simulink model "gm_sampleModel1810_sub"  (R2023a)
settings: Solver=VariableStepAuto  StartTime=0.0  StopTime=10.0  RelTol=1e-3
libraries: simulink x4, hdlsllib x2
settings Model: Creator=user1  LastModifiedBy=user1
settings OptimizationCC: BlockReduction=off  ConditionallyExecuteInputs=off
settings DebuggingCC: InheritedTsInSrcMsg=none

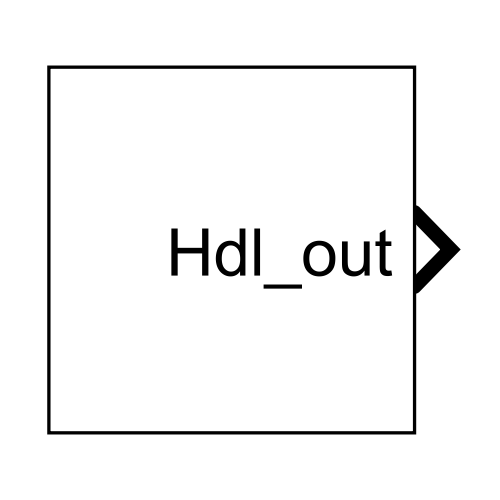
[thumbnail: Simulink's stored preview of the top-level diagram]
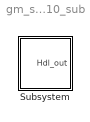
== system gm_sampleModel1810_sub ==
  Subsystem : Subsystem

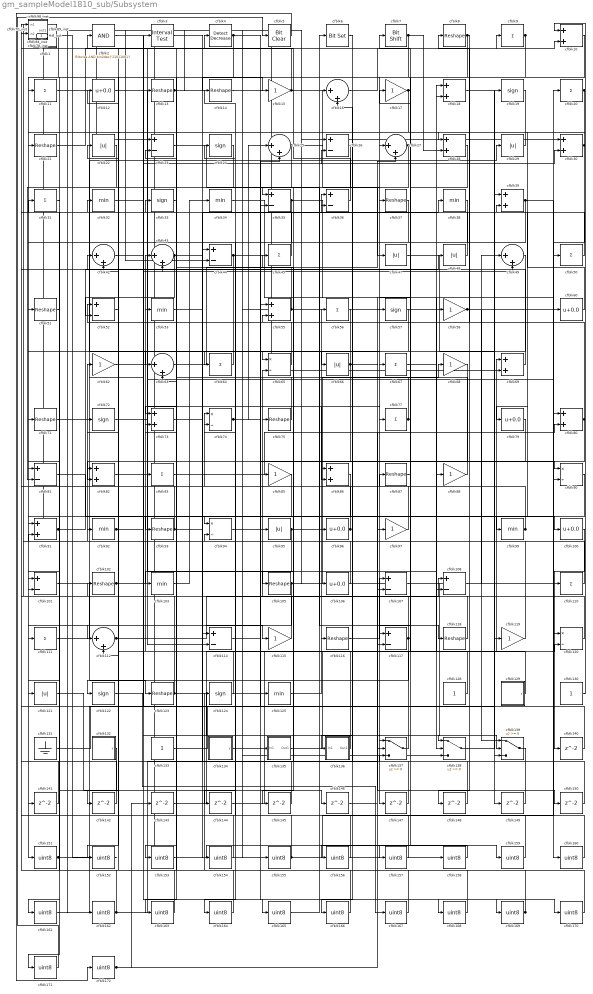
== system gm_sampleModel1810_sub/Subsystem ==
  cfblk1 : Subsystem  mask(Detect Rise Nonnegative){vinit=double(0), InputProcessing=Elements as channels (sample based), OutDataTypeStr=uint8}
      mask prompts: vinit "Simulink:masks:InitialCondition_MP"; InputProcessing "Simulink:masks:InputProcessing_MP"; OutDataTypeStr "Simulink:masks:OutputDataType_MP"
      mask help: Simulink:masks:DetectRiseNonnegative_MD
      mask init:
      | InputProcessing = 'Elements as channels (sample based)';
      | OutDataTypeStr = 'uint8';
      | vinit = double(0);
      mask TypeOptions InputProcessing: Simulink:masks:ColumnsAsChannelsFrameBased | Simulink:masks:ElementsAsChannelsSampleBased
      mask TypeOptions OutDataTypeStr: Simulink:masks:uint8 | Simulink:masks:boolean
      mask Display: fprintf('U >= 0\n&  NOT\nU/z >= 0')
  cfblk{10,18,28,30,39,55,69,73,80,82,86,91} (12 alike) : Sum  OutDataTypeStr=uint8
  cfblk{12,60,79,96,100,106} (6 alike) : Bias  Bias=0.0  SaturateOnIntegerOverflow=off
  cfblk{23,26,35..36,44,52,81,101,107..108,114,117} (12 alike) : Sum  Inputs=+-  OutDataTypeStr=uint8
  cfblk{8,13..14,21,37,51,71,75,87,93,102,105,116,118,123} (15 alike) : Reshape
  cfblk{32,34,38,53,92,99,103,125} (8 alike) : MinMax  OutDataTypeStr=uint8
  cfblk{9,11,20,31,45,50,56,64,67,77,83,110..111} (13 alike) : Sum  Inputs=+  OutDataTypeStr=uint8
  cfblk{16,25,27,42..43,49,63,112} (8 alike) : Sum  Inputs=|++  OutDataTypeStr=uint8
  cfblk113_inst : Subsystem
  cfblk{15,17,58,62,68,85,88,97,115,119} (10 alike) : Gain  OutDataTypeStr=uint8
  cfblk{65,74,90,94,120} (5 alike) : Product  Inputs=*/  OutDataTypeStr=uint8  RndMeth=Zero  SaturateOnIntegerOverflow=on
  cfblk{22,29,47..48,66,95,121} (7 alike) : Abs  OutDataTypeStr=uint8  SaturateOnIntegerOverflow=off
  cfblk{19,24,33,57,72,122,124} (7 alike) : Signum
  cfblk128 : Constant  OutDataTypeStr=uint8  SampleTime=-1
  cfblk129 : Subsystem  mask(Counter Limited){uplimit=double(7), tsamp=double(-1)}
      mask prompts: uplimit "Simulink:masks:UpperLimit_MP"; tsamp "Simulink:masks:SampleTime_MP"
      mask help: Simulink:masks:CounterLimited_MD
      mask init:
      | nbits = double(8);
      | tsamp = double(-1);
      | uplimit = double(7);
  cfblk130 : Constant  OutDataTypeStr=uint8  SampleTime=-1
  cfblk131 : Ground
  cfblk132 : Subsystem  mask(Counter Free-Running){NumBits=double(16), tsamp=double(-1)}
      mask prompts: NumBits "Simulink:masks:NumberOfBits_MP"; tsamp "Simulink:masks:SampleTime_MP"
      mask help: Simulink:masks:CounterFreeRunning_MD
  cfblk133 : Constant  OutDataTypeStr=uint8  SampleTime=-1
  cfblk134 : Subsystem  mask(Counter Limited){uplimit=double(7), tsamp=double(-1)}
      mask prompts: uplimit "Simulink:masks:UpperLimit_MP"; tsamp "Simulink:masks:SampleTime_MP"
      mask help: Simulink:masks:CounterLimited_MD
      mask init:
      | nbits = double(8);
      | tsamp = double(-1);
      | uplimit = double(7);
  cfblk135 : Subsystem
  cfblk136 : Subsystem
  cfblk137 : Switch  OutDataTypeStr=uint8  SaturateOnIntegerOverflow=off  InputSameDT=off
  cfblk138 : Switch  OutDataTypeStr=uint8  SaturateOnIntegerOverflow=off  InputSameDT=off
  cfblk139 : Switch  OutDataTypeStr=uint8  SaturateOnIntegerOverflow=off  InputSameDT=off
  cfblk{140..150} (11 alike) : Delay  SampleTime=1
  cfblk{151..172} (22 alike) : DataTypeConversion  OutDataTypeStr=uint8  SaturateOnIntegerOverflow=off  RndMeth=Floor
  cfblk2 : simulink/Logic and Bit Operations/Bitwise Operator  logicop=AND  UseBitMask=on  BitMask=bin2dec('11011001')  BitMaskRealWorld=Stored Integer
      settings: LibrarySourceBlock=|
      | hdlsllib/Logic and Bit
      | Operations/Bitwise
      | Operator
  cfblk3 : hdlsllib/Logic and Bit Operations/Interval Test  IntervalClosedRight=on  uplimit=0.5  IntervalClosedLeft=on  lowlimit=-0.5  OutDataTypeStr=uint8
  cfblk4 : simulink/Logic and Bit Operations/Detect Decrease  vinit=0.0  OutDataTypeStr=uint8
      settings: LibrarySourceBlock=|
      | hdlsllib/Logic and Bit
      | Operations/Detect
      | Decrease
  cfblk41_inst : Subsystem
  cfblk46_inst : Subsystem
  cfblk5 : simulink/Logic and Bit Operations/Bit Clear  iBit=0
      settings: LibrarySourceBlock=|
      | hdlsllib/Logic and Bit
      | Operations/Bit Clear
  cfblk54_inst : Subsystem
  cfblk59_inst : Subsystem
  cfblk6 : simulink/Logic and Bit Operations/Bit Set  iBit=0
      settings: LibrarySourceBlock=|
      | hdlsllib/Logic and Bit
      | Operations/Bit Set
  cfblk61_inst : Subsystem
  cfblk7 : hdlsllib/Logic and Bit Operations/Bit Shift  mode=Shift Left Logical  N=0
  cfblk70_inst : Subsystem
  cfblk78_inst : Subsystem
  cfblk84_inst : Subsystem
  cfblk89_inst : Subsystem
  cfblk98_inst : Subsystem
  Hdl_out : Outport  OutDataTypeStr=uint8  SampleTime=1
  wires:
  cfblk1/1(Y) -> cfblk151/1
  cfblk10/1 -> cfblk147/1
  cfblk100/1 -> cfblk140/1
  cfblk101/1 -> cfblk123/1
  cfblk102/1 -> cfblk114/2, cfblk10/2
  cfblk103/1 -> cfblk34/1
  cfblk105/1 -> cfblk68/1, cfblk141/1
  cfblk106/1 -> cfblk84_inst/1(in1)
  cfblk107/1 -> cfblk139/2
  cfblk108/1 -> cfblk49/1
  cfblk11/1 -> cfblk67/1
  cfblk110/1 -> cfblk65/2
  cfblk111/1 -> cfblk29/1
  cfblk112/1 -> cfblk108/1, cfblk115/1
  cfblk113_inst/1(out1) -> cfblk44/2, cfblk138/3
  cfblk114/1 -> cfblk120/2
  cfblk115/1 -> cfblk14/1
  cfblk116/1 -> cfblk107/1
  cfblk117/1 -> cfblk78_inst/1(in1), cfblk122/1
  cfblk118/1 -> cfblk113_inst/1(in1)
  cfblk119/1 -> cfblk62/1
  cfblk12/1 -> cfblk107/2
  cfblk120/1 -> cfblk75/1
  cfblk121/1 -> cfblk146/1
  cfblk122/1 -> cfblk167/1
  cfblk123/1 -> cfblk78_inst/2(in2), cfblk139/3, cfblk138/1
  cfblk124/1 -> cfblk43/1
  cfblk125/1 -> cfblk56/1
  cfblk128/1 -> cfblk17/1
  cfblk129/1(y) -> cfblk92/1
  cfblk13/1 -> cfblk15/1, cfblk77/1
  cfblk130/1 -> cfblk10/1
  cfblk131/1 -> cfblk25/2
  cfblk132/1(y) -> cfblk161/1
  cfblk133/1 -> cfblk19/1
  cfblk134/1(y) -> cfblk116/1
  cfblk135/1(Out1) -> cfblk18/2
  cfblk136/1(Out1) -> cfblk74/1
  cfblk137/1 -> cfblk53/1
  cfblk138/1 -> cfblk120/1
  cfblk139/1 -> cfblk137/3
  cfblk14/1 -> cfblk90/1
  cfblk140/1 -> cfblk84_inst/2(in2)
  cfblk141/1 -> cfblk70_inst/2(in2)
  cfblk142/1 -> cfblk46_inst/2(in2)
  cfblk143/1 -> cfblk69/1
  cfblk144/1 -> cfblk39/1
  cfblk145/1 -> cfblk52/1
  cfblk146/1 -> cfblk80/2
  cfblk147/1 -> cfblk55/2
  cfblk148/1 -> cfblk16/2
  cfblk149/1 -> cfblk36/1
  cfblk15/1 -> cfblk59_inst/2(in2), cfblk37/1
  cfblk150/1 -> cfblk44/1
  cfblk151/1 -> cfblk106/1, cfblk3/1
  cfblk152/1 -> cfblk1/1(U)
  cfblk153/1 -> cfblk159/1
  cfblk154/1 -> cfblk33/1
  cfblk155/1 -> cfblk94/2, cfblk50/1
  cfblk156/1 -> cfblk61_inst/1(in1)
  cfblk157/1 -> cfblk61_inst/2(in2)
  cfblk158/1 -> cfblk156/1
  cfblk159/1 -> cfblk54_inst/1(in1)
  cfblk16/1 -> cfblk9/1
  cfblk160/1 -> cfblk54_inst/2(in2)
  cfblk161/1 -> cfblk95/1
  cfblk162/1 -> cfblk98_inst/2(in2), cfblk91/2, cfblk137/2, cfblk31/1
  cfblk163/1 -> cfblk89_inst/1(in1)
  cfblk164/1 -> cfblk89_inst/2(in2)
  cfblk165/1 -> cfblk6/1
  cfblk166/1 -> cfblk124/1
  cfblk167/1 -> cfblk2/1
  cfblk168/1 -> cfblk102/1
  cfblk169/1 -> cfblk73/2, cfblk22/1
  cfblk17/1 -> cfblk93/1, cfblk157/1
  cfblk170/1 -> cfblk32/1
  cfblk171/1 -> cfblk5/1
  cfblk172/1 -> cfblk117/2, cfblk143/1
  cfblk18/1 -> cfblk149/1
  cfblk19/1 -> cfblk28/1
  cfblk2/1 -> cfblk168/1
  cfblk20/1 -> cfblk79/1, cfblk101/2
  cfblk21/1 -> cfblk4/1
  cfblk22/1 -> cfblk171/1
  cfblk23/1 -> cfblk96/1
  cfblk24/1 -> cfblk81/1
  cfblk25/1 -> cfblk81/2, cfblk47/1
  cfblk26/1 -> cfblk105/1
  cfblk27/1 -> cfblk35/1, cfblk112/2
  cfblk28/1 -> cfblk57/1
  cfblk29/1 -> cfblk21/1
  cfblk3/1 -> cfblk154/1
  cfblk30/1 -> cfblk27/1, cfblk90/2
  cfblk31/1 -> cfblk101/1
  cfblk32/1 -> cfblk169/1
  cfblk33/1 -> cfblk153/1
  cfblk34/1 -> cfblk97/1
  cfblk35/1 -> cfblk51/1, cfblk138/2
  cfblk36/1 -> cfblk46_inst/1(in1)
  cfblk37/1 -> cfblk103/1
  cfblk38/1 -> cfblk65/1
  cfblk39/1 -> cfblk80/1, cfblk94/1, cfblk99/1
  cfblk4/1 -> cfblk91/1, cfblk170/1
  cfblk41_inst/1(out1) -> cfblk13/1
  cfblk42/1 -> cfblk165/1
  cfblk43/1 -> cfblk52/2, cfblk108/2
  cfblk44/1 -> cfblk71/1, cfblk160/1
  cfblk45/1 -> cfblk59_inst/1(in1)
  cfblk46_inst/1(out1) -> cfblk69/2
  cfblk47/1 -> cfblk119/1
  cfblk48/1 -> cfblk12/1
  cfblk49/1 -> cfblk145/1
  cfblk5/1 -> cfblk172/1
  cfblk50/1 -> cfblk39/2
  cfblk51/1 -> cfblk121/1
  cfblk52/1 -> cfblk112/1
  cfblk53/1 -> cfblk114/1
  cfblk54_inst/1(out1) -> cfblk158/1
  cfblk55/1 -> cfblk41_inst/2(in2), cfblk118/1
  cfblk56/1 -> cfblk164/1
  cfblk57/1 -> cfblk66/1
  cfblk58/1 -> cfblk60/1, cfblk139/1
  cfblk59_inst/1(out1) -> cfblk125/1
  cfblk6/1 -> cfblk166/1
  cfblk60/1 -> cfblk36/2
  cfblk61_inst/1(out1) -> cfblk155/1
  cfblk62/1 -> cfblk86/2
  cfblk63/1 -> cfblk27/2
  cfblk64/1 -> cfblk63/1
  cfblk65/1 -> cfblk42/1
  cfblk66/1 -> cfblk82/2, cfblk150/1, cfblk64/1
  cfblk67/1 -> cfblk88/1
  cfblk68/1 -> cfblk142/1
  cfblk69/1 -> cfblk70_inst/1(in1)
  cfblk7/1 -> cfblk82/1, cfblk28/2
  cfblk70_inst/1(out1) -> cfblk23/1, cfblk16/1
  cfblk71/1 -> cfblk26/2
  cfblk72/1 -> cfblk20/1
  cfblk73/1 -> cfblk38/1
  cfblk74/1 -> cfblk35/2, cfblk25/1
  cfblk75/1 -> cfblk24/1
  cfblk77/1 -> cfblk23/2, cfblk113_inst/2(in2)
  cfblk78_inst/1(out1) -> cfblk98_inst/1(in1), cfblk110/1
  cfblk79/1 -> cfblk86/1
  cfblk8/1 -> cfblk117/1, cfblk148/1
  cfblk80/1 -> cfblk8/1, cfblk136/1(In1), cfblk45/1
  cfblk81/1 -> cfblk100/1
  cfblk82/1 -> cfblk135/1(In1)
  cfblk83/1 -> cfblk18/1
  cfblk84_inst/1(out1) -> cfblk58/1
  cfblk85/1 -> cfblk152/1
  cfblk86/1 -> cfblk111/1
  cfblk87/1 -> cfblk7/1
  cfblk88/1 -> cfblk55/1
  cfblk89_inst/1(out1) -> cfblk162/1
  cfblk9/1 -> cfblk73/1, cfblk11/1
  cfblk90/1 -> cfblk144/1
  cfblk91/1 -> cfblk48/1, Hdl_out/1
  cfblk92/1 -> cfblk72/1, cfblk49/2, cfblk43/2, cfblk137/1
  cfblk93/1 -> cfblk41_inst/1(in1), cfblk85/1
  cfblk94/1 -> cfblk26/1
  cfblk95/1 -> cfblk30/2, cfblk163/1
  cfblk96/1 -> cfblk63/2, cfblk74/2
  cfblk97/1 -> cfblk42/2
  cfblk98_inst/1(out1) -> cfblk30/1
  cfblk99/1 -> cfblk87/1, cfblk83/1

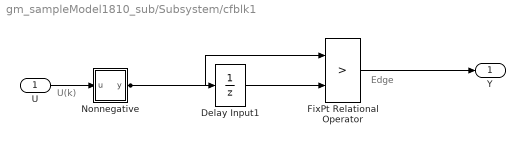
== system gm_sampleModel1810_sub/Subsystem/cfblk1 ==
  note: U(k)
  note: Edge
  U : Inport  OutDataTypeStr=uint8  SampleTime=1
  Delay Input1 : UnitDelay  Description=Store in Global RAM  DisableCoverage=on  InitialCondition=vinit  SampleTime=-1  HasFrameUpgradeWarning=on
  FixPt Relational Operator : RelationalOperator  Operator=>  OutDataTypeStr=fixdt(0, 8)  ZeroCross=off  InputSameDT=off
  Nonnegative : Subsystem  mask(Compare To Zero){relop=>=, OutDataTypeStr=boolean, ZeroCross=off}
      mask prompts: relop "Simulink:masks:Operator_MP"; OutDataTypeStr "Simulink:masks:OutputDataType_MP"; ZeroCross "Simulink:masks:EnableZerocrossingDetection_MP"
      mask help: Simulink:masks:CompareToZero_MD
      mask init:
      | OutDataTypeStr = 'boolean';
      | ZeroCross = 'off';
      | blkName = 'sampleModel1810_sub/Subsystem/cfblk1/Nonnegative';
      | relop = '>=';
      | setValue = 'boolean';
      mask TypeOptions relop: == | ~= | < | <= | >= | >
      mask TypeOptions OutDataTypeStr: Simulink:masks:uint8 | Simulink:masks:boolean
      mask Callback ZeroCross: sl('zeroCrossEnable', gcbh);
      mask Display: disp([relop,' 0'])
  Y : Outport  SampleTime=1
  wires:
  U/1 -> Nonnegative/1(u)
  Delay Input1/1 -> FixPt Relational Operator/2
  FixPt Relational Operator/1 -> Y/1
  Nonnegative/1(y) -> FixPt Relational Operator/1, Delay Input1/1

== system gm_sampleModel1810_sub/Subsystem/cfblk113_inst ==
  in1 : Inport  OutDataTypeStr=uint8  SampleTime=1
  in2 : Inport  Port=2  OutDataTypeStr=uint8  SampleTime=1
  mul_cfblk113_dotp_mulcomp : Product  Inputs=**  OutDataTypeStr=uint8  SampleTime=1
  out1 : Outport  OutDataTypeStr=uint8  SampleTime=1
  wires:
  in1/1 -> mul_cfblk113_dotp_mulcomp/1
  in2/1 -> mul_cfblk113_dotp_mulcomp/2
  mul_cfblk113_dotp_mulcomp/1 -> out1/1

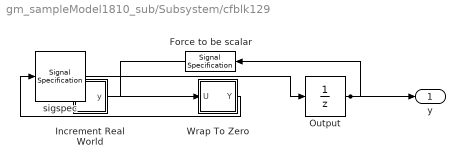
== system gm_sampleModel1810_sub/Subsystem/cfblk129 ==
  Force to be scalar : SignalSpecification  DisableCoverage=on  Dimensions=1
  Increment Real World : Subsystem  mask(Real World Value Increment){}
      mask help: Simulink:masks:RealWorldValueIncrement_MD
      mask Display: disp('V++')
  Output : UnitDelay  InitialCondition=0.0  SampleTime=tsamp  HasFrameUpgradeWarning=on
  Wrap To Zero : Subsystem  mask(Wrap To Zero){Threshold=double(7)}
      mask prompts: Threshold "Simulink:masks:Threshold_MP"
      mask help: Simulink:masks:WrapToZero_MD
  sigspec : SignalSpecification  OutDataTypeStr=uint8  Dimensions=1
  y : Outport  SampleTime=1
  wires:
  Force to be scalar/1 -> Increment Real World/1(u)
  Increment Real World/1(y) -> Wrap To Zero/1(U)
  Output/1 -> Force to be scalar/1, y/1
  Wrap To Zero/1(Y) -> sigspec/1
  sigspec/1 -> Output/1

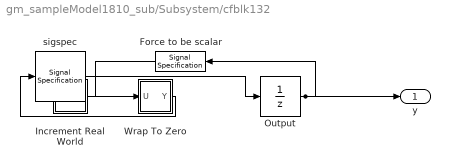
== system gm_sampleModel1810_sub/Subsystem/cfblk132 ==
  Force to be scalar : SignalSpecification  DisableCoverage=on  Dimensions=1
  Increment Real World : Subsystem  mask(Real World Value Increment){}
      mask help: Simulink:masks:RealWorldValueIncrement_MD
      mask Display: disp('V++')
  Output : UnitDelay  InitialCondition=0.0  SampleTime=tsamp  HasFrameUpgradeWarning=on
  Wrap To Zero : Subsystem  mask(Wrap To Zero){Threshold=double(65535)}
      mask prompts: Threshold "Simulink:masks:Threshold_MP"
      mask help: Simulink:masks:WrapToZero_MD
  sigspec : SignalSpecification  OutDataTypeStr=uint16  Dimensions=1
  y : Outport  SampleTime=1
  wires:
  Force to be scalar/1 -> Increment Real World/1(u)
  Increment Real World/1(y) -> Wrap To Zero/1(U)
  Output/1 -> Force to be scalar/1, y/1
  Wrap To Zero/1(Y) -> sigspec/1
  sigspec/1 -> Output/1

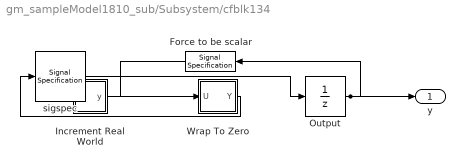
== system gm_sampleModel1810_sub/Subsystem/cfblk134 ==
  Force to be scalar : SignalSpecification  DisableCoverage=on  Dimensions=1
  Increment Real World : Subsystem  mask(Real World Value Increment){}
      mask help: Simulink:masks:RealWorldValueIncrement_MD
      mask Display: disp('V++')
  Output : UnitDelay  InitialCondition=0.0  SampleTime=tsamp  HasFrameUpgradeWarning=on
  Wrap To Zero : Subsystem  mask(Wrap To Zero){Threshold=double(7)}
      mask prompts: Threshold "Simulink:masks:Threshold_MP"
      mask help: Simulink:masks:WrapToZero_MD
  sigspec : SignalSpecification  OutDataTypeStr=uint8  Dimensions=1
  y : Outport  SampleTime=1
  wires:
  Force to be scalar/1 -> Increment Real World/1(u)
  Increment Real World/1(y) -> Wrap To Zero/1(U)
  Output/1 -> Force to be scalar/1, y/1
  Wrap To Zero/1(Y) -> sigspec/1
  sigspec/1 -> Output/1

== system gm_sampleModel1810_sub/Subsystem/cfblk135 ==
  In1 : Inport  OutDataTypeStr=uint8  PortDimensions=1  SampleTime=1
  Out1 : Outport  SampleTime=1
  wires:
  In1/1 -> Out1/1

== system gm_sampleModel1810_sub/Subsystem/cfblk136 ==
  In1 : Inport  OutDataTypeStr=uint8  PortDimensions=1  SampleTime=1
  Out1 : Outport  SampleTime=1
  wires:
  In1/1 -> Out1/1

== system gm_sampleModel1810_sub/Subsystem/cfblk41_inst ==
  in1 : Inport  OutDataTypeStr=uint8  SampleTime=1
  in2 : Inport  Port=2  OutDataTypeStr=uint8  SampleTime=1
  mul_cfblk41_dotp_mulcomp : Product  Inputs=**  OutDataTypeStr=uint8  SampleTime=1
  out1 : Outport  OutDataTypeStr=uint8  SampleTime=1
  wires:
  in1/1 -> mul_cfblk41_dotp_mulcomp/1
  in2/1 -> mul_cfblk41_dotp_mulcomp/2
  mul_cfblk41_dotp_mulcomp/1 -> out1/1

== system gm_sampleModel1810_sub/Subsystem/cfblk46_inst ==
  in1 : Inport  OutDataTypeStr=uint8  SampleTime=1
  in2 : Inport  Port=2  OutDataTypeStr=uint8  SampleTime=1
  mul_cfblk46_dotp_mulcomp : Product  Inputs=**  OutDataTypeStr=uint8  SampleTime=1
  out1 : Outport  OutDataTypeStr=uint8  SampleTime=1
  wires:
  in1/1 -> mul_cfblk46_dotp_mulcomp/1
  in2/1 -> mul_cfblk46_dotp_mulcomp/2
  mul_cfblk46_dotp_mulcomp/1 -> out1/1

== system gm_sampleModel1810_sub/Subsystem/cfblk54_inst ==
  in1 : Inport  OutDataTypeStr=uint8  SampleTime=1
  in2 : Inport  Port=2  OutDataTypeStr=uint8  SampleTime=1
  mul_cfblk54_dotp_mulcomp : Product  Inputs=**  OutDataTypeStr=uint8  SampleTime=1
  out1 : Outport  OutDataTypeStr=uint8  SampleTime=1
  wires:
  in1/1 -> mul_cfblk54_dotp_mulcomp/1
  in2/1 -> mul_cfblk54_dotp_mulcomp/2
  mul_cfblk54_dotp_mulcomp/1 -> out1/1

== system gm_sampleModel1810_sub/Subsystem/cfblk59_inst ==
  in1 : Inport  OutDataTypeStr=uint8  SampleTime=1
  in2 : Inport  Port=2  OutDataTypeStr=uint8  SampleTime=1
  mul_cfblk59_dotp_mulcomp : Product  Inputs=**  OutDataTypeStr=uint8  SampleTime=1
  out1 : Outport  OutDataTypeStr=uint8  SampleTime=1
  wires:
  in1/1 -> mul_cfblk59_dotp_mulcomp/1
  in2/1 -> mul_cfblk59_dotp_mulcomp/2
  mul_cfblk59_dotp_mulcomp/1 -> out1/1

== system gm_sampleModel1810_sub/Subsystem/cfblk61_inst ==
  in1 : Inport  OutDataTypeStr=uint8  SampleTime=1
  in2 : Inport  Port=2  OutDataTypeStr=uint8  SampleTime=1
  mul_cfblk61_dotp_mulcomp : Product  Inputs=**  OutDataTypeStr=uint8  SampleTime=1
  out1 : Outport  OutDataTypeStr=uint8  SampleTime=1
  wires:
  in1/1 -> mul_cfblk61_dotp_mulcomp/1
  in2/1 -> mul_cfblk61_dotp_mulcomp/2
  mul_cfblk61_dotp_mulcomp/1 -> out1/1

== system gm_sampleModel1810_sub/Subsystem/cfblk70_inst ==
  in1 : Inport  OutDataTypeStr=uint8  SampleTime=1
  in2 : Inport  Port=2  OutDataTypeStr=uint8  SampleTime=1
  mul_cfblk70_dotp_mulcomp : Product  Inputs=**  OutDataTypeStr=uint8  SampleTime=1
  out1 : Outport  OutDataTypeStr=uint8  SampleTime=1
  wires:
  in1/1 -> mul_cfblk70_dotp_mulcomp/1
  in2/1 -> mul_cfblk70_dotp_mulcomp/2
  mul_cfblk70_dotp_mulcomp/1 -> out1/1

== system gm_sampleModel1810_sub/Subsystem/cfblk78_inst ==
  in1 : Inport  OutDataTypeStr=uint8  SampleTime=1
  in2 : Inport  Port=2  OutDataTypeStr=uint8  SampleTime=1
  mul_cfblk78_dotp_mulcomp : Product  Inputs=**  OutDataTypeStr=uint8  SampleTime=1
  out1 : Outport  OutDataTypeStr=uint8  SampleTime=1
  wires:
  in1/1 -> mul_cfblk78_dotp_mulcomp/1
  in2/1 -> mul_cfblk78_dotp_mulcomp/2
  mul_cfblk78_dotp_mulcomp/1 -> out1/1

== system gm_sampleModel1810_sub/Subsystem/cfblk84_inst ==
  in1 : Inport  OutDataTypeStr=uint8  SampleTime=1
  in2 : Inport  Port=2  OutDataTypeStr=uint8  SampleTime=1
  mul_cfblk84_dotp_mulcomp : Product  Inputs=**  OutDataTypeStr=uint8  SampleTime=1
  out1 : Outport  OutDataTypeStr=uint8  SampleTime=1
  wires:
  in1/1 -> mul_cfblk84_dotp_mulcomp/1
  in2/1 -> mul_cfblk84_dotp_mulcomp/2
  mul_cfblk84_dotp_mulcomp/1 -> out1/1

== system gm_sampleModel1810_sub/Subsystem/cfblk89_inst ==
  in1 : Inport  OutDataTypeStr=uint8  SampleTime=1
  in2 : Inport  Port=2  OutDataTypeStr=uint8  SampleTime=1
  mul_cfblk89_dotp_mulcomp : Product  Inputs=**  OutDataTypeStr=uint8  SampleTime=1
  out1 : Outport  OutDataTypeStr=uint8  SampleTime=1
  wires:
  in1/1 -> mul_cfblk89_dotp_mulcomp/1
  in2/1 -> mul_cfblk89_dotp_mulcomp/2
  mul_cfblk89_dotp_mulcomp/1 -> out1/1

== system gm_sampleModel1810_sub/Subsystem/cfblk98_inst ==
  in1 : Inport  OutDataTypeStr=uint8  SampleTime=1
  in2 : Inport  Port=2  OutDataTypeStr=uint8  SampleTime=1
  mul_cfblk98_dotp_mulcomp : Product  Inputs=**  OutDataTypeStr=uint8  SampleTime=1
  out1 : Outport  OutDataTypeStr=uint8  SampleTime=1
  wires:
  in1/1 -> mul_cfblk98_dotp_mulcomp/1
  in2/1 -> mul_cfblk98_dotp_mulcomp/2
  mul_cfblk98_dotp_mulcomp/1 -> out1/1

== system gm_sampleModel1810_sub/Subsystem/cfblk1/Nonnegative ==
  u : Inport  OutDataTypeStr=uint8  SampleTime=1
  Compare : RelationalOperator  OutDataTypeStr=boolean  ZeroCross=off
  Constant : Constant  DisableCoverage=on  Value=0  OutDataTypeStr=Inherit: Inherit via back propagation  SampleTime=-1  PreserveConstantTs=on
  y : Outport  SampleTime=1
  wires:
  u/1 -> Compare/1
  Compare/1 -> y/1
  Constant/1 -> Compare/2

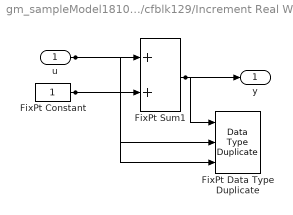
== system gm_sampleModel1810_sub/Subsystem/cfblk129/Increment Real World ==
  u : Inport  OutDataTypeStr=uint8  SampleTime=1
  FixPt Constant : Constant  DisableCoverage=on  OutDataTypeStr=Inherit: Inherit via back propagation  SampleTime=-1
  FixPt Data Type Duplicate : DataTypeDuplicate  DisableCoverage=on  NumInputPorts=3
  FixPt Sum1 : Sum  InputSameDT=on  OutDataTypeStr=Inherit: Inherit via back propagation  LockScale=on
  y : Outport  SampleTime=1
  wires:
  u/1 -> FixPt Sum1/1, FixPt Data Type Duplicate/2
  FixPt Constant/1 -> FixPt Sum1/2, FixPt Data Type Duplicate/3
  FixPt Sum1/1 -> FixPt Data Type Duplicate/1, y/1

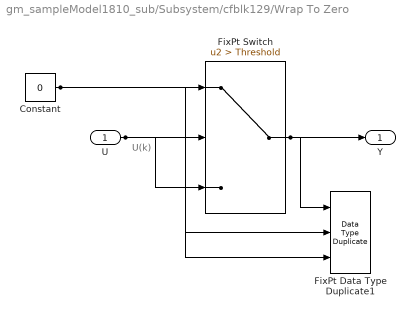
== system gm_sampleModel1810_sub/Subsystem/cfblk129/Wrap To Zero ==
  note: U(k)
  U : Inport  OutDataTypeStr=uint8  SampleTime=1
  Constant : Constant  DisableCoverage=on  Value=0  OutDataTypeStr=Inherit: Inherit via back propagation  SampleTime=-1
  FixPt Data Type Duplicate1 : DataTypeDuplicate  DisableCoverage=on  NumInputPorts=3
  FixPt Switch : Switch  Criteria=u2 > Threshold  Threshold=Threshold  OutDataTypeStr=Inherit: Inherit via back propagation  ZeroCross=off  SaturateOnIntegerOverflow=off  InputSameDT=off
  Y : Outport  SampleTime=1
  wires:
  U/1 -> FixPt Switch/3, FixPt Switch/2, FixPt Data Type Duplicate1/2
  Constant/1 -> FixPt Switch/1, FixPt Data Type Duplicate1/3
  FixPt Switch/1 -> FixPt Data Type Duplicate1/1, Y/1

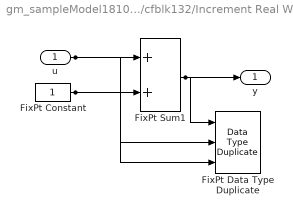
== system gm_sampleModel1810_sub/Subsystem/cfblk132/Increment Real World ==
  u : Inport  OutDataTypeStr=uint16  SampleTime=1
  FixPt Constant : Constant  DisableCoverage=on  OutDataTypeStr=Inherit: Inherit via back propagation  SampleTime=-1
  FixPt Data Type Duplicate : DataTypeDuplicate  DisableCoverage=on  NumInputPorts=3
  FixPt Sum1 : Sum  InputSameDT=on  OutDataTypeStr=Inherit: Inherit via back propagation  LockScale=on
  y : Outport  SampleTime=1
  wires:
  u/1 -> FixPt Sum1/1, FixPt Data Type Duplicate/2
  FixPt Constant/1 -> FixPt Sum1/2, FixPt Data Type Duplicate/3
  FixPt Sum1/1 -> FixPt Data Type Duplicate/1, y/1

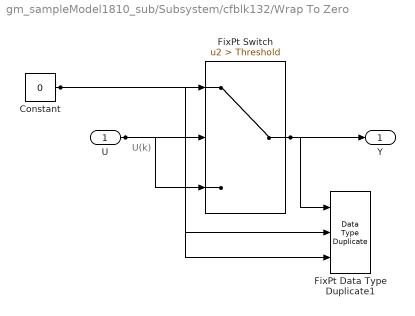
== system gm_sampleModel1810_sub/Subsystem/cfblk132/Wrap To Zero ==
  note: U(k)
  U : Inport  OutDataTypeStr=uint16  SampleTime=1
  Constant : Constant  DisableCoverage=on  Value=0  OutDataTypeStr=Inherit: Inherit via back propagation  SampleTime=-1
  FixPt Data Type Duplicate1 : DataTypeDuplicate  DisableCoverage=on  NumInputPorts=3
  FixPt Switch : Switch  Criteria=u2 > Threshold  Threshold=Threshold  OutDataTypeStr=Inherit: Inherit via back propagation  ZeroCross=off  SaturateOnIntegerOverflow=off  InputSameDT=off
  Y : Outport  SampleTime=1
  wires:
  U/1 -> FixPt Switch/3, FixPt Switch/2, FixPt Data Type Duplicate1/2
  Constant/1 -> FixPt Switch/1, FixPt Data Type Duplicate1/3
  FixPt Switch/1 -> FixPt Data Type Duplicate1/1, Y/1

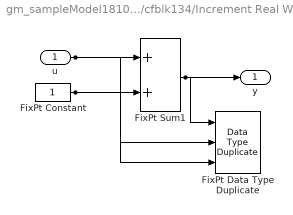
== system gm_sampleModel1810_sub/Subsystem/cfblk134/Increment Real World ==
  u : Inport  OutDataTypeStr=uint8  SampleTime=1
  FixPt Constant : Constant  DisableCoverage=on  OutDataTypeStr=Inherit: Inherit via back propagation  SampleTime=-1
  FixPt Data Type Duplicate : DataTypeDuplicate  DisableCoverage=on  NumInputPorts=3
  FixPt Sum1 : Sum  InputSameDT=on  OutDataTypeStr=Inherit: Inherit via back propagation  LockScale=on
  y : Outport  SampleTime=1
  wires:
  u/1 -> FixPt Sum1/1, FixPt Data Type Duplicate/2
  FixPt Constant/1 -> FixPt Sum1/2, FixPt Data Type Duplicate/3
  FixPt Sum1/1 -> FixPt Data Type Duplicate/1, y/1

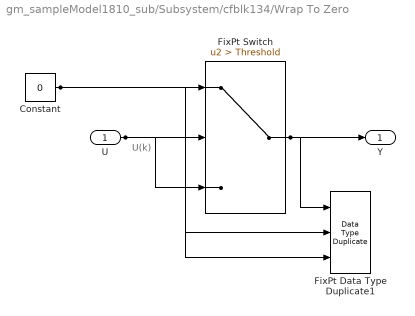
== system gm_sampleModel1810_sub/Subsystem/cfblk134/Wrap To Zero ==
  note: U(k)
  U : Inport  OutDataTypeStr=uint8  SampleTime=1
  Constant : Constant  DisableCoverage=on  Value=0  OutDataTypeStr=Inherit: Inherit via back propagation  SampleTime=-1
  FixPt Data Type Duplicate1 : DataTypeDuplicate  DisableCoverage=on  NumInputPorts=3
  FixPt Switch : Switch  Criteria=u2 > Threshold  Threshold=Threshold  OutDataTypeStr=Inherit: Inherit via back propagation  ZeroCross=off  SaturateOnIntegerOverflow=off  InputSameDT=off
  Y : Outport  SampleTime=1
  wires:
  U/1 -> FixPt Switch/3, FixPt Switch/2, FixPt Data Type Duplicate1/2
  Constant/1 -> FixPt Switch/1, FixPt Data Type Duplicate1/3
  FixPt Switch/1 -> FixPt Data Type Duplicate1/1, Y/1
